simulink model "crazy_ride"  (R2016a)
settings: Solver=VariableStepAuto  StartTime=0.0  StopTime=10.0  RelTol=1e-3
settings Model: Creator=mgreiff  LastModifiedBy=mgreiff

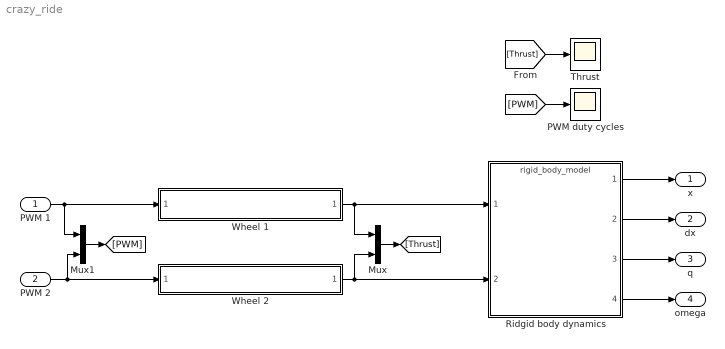
== system crazy_ride ==
  PWM 1 : Inport
  PWM 2 : Inport  Port=2
  Mux : Mux  Inputs=2
  Mux1 : Mux  Inputs=2
  PWM duty cycles : Scope
  Ridgid body dynamics : ModelReference  ModelNameDialog=rigid_body_model.slx  SimulationMode=Normal  ModelReferenceVersion=1.165
  Thrust : Scope
  Wheel 1 : ModelReference  ModelNameDialog=wheel_model.slx  SimulationMode=Normal  ModelReferenceVersion=1.6
  Wheel 2 : ModelReference  ModelNameDialog=wheel_model.slx  SimulationMode=Normal  ModelReferenceVersion=1.6
  x : Outport
  dx : Outport  Port=2
  q : Outport  Port=3
  omega : Outport  Port=4
  wires:
  Wheel 1/1 -> Mux/1, Ridgid body dynamics/1
  Wheel 2/1 -> Mux/2, Ridgid body dynamics/2
  PWM 1/1 -> Mux1/1, Wheel 1/1
  PWM 2/1 -> Mux1/2, Wheel 2/1
  Mux/1 -> [Thrust]
  Mux1/1 -> [PWM]
  Ridgid body dynamics/2 -> dx/1
  Ridgid body dynamics/3 -> q/1
  Ridgid body dynamics/4 -> omega/1
  Ridgid body dynamics/1 -> x/1
  [Thrust] -> Thrust/1
  [PWM] -> PWM duty cycles/1
